simulink model "ex6_dvbs_chain_v2"  (R2022a)
settings: Solver=VariableStepAuto  StartTime=0.0  StopTime=1  RelTol=1e-3
values from neighbouring files (symbols this model uses):
  M = 4    [ex6_parameters.m]
  PS_beta = 0.35    [ex6_parameters.m]
  PS_osf = 10    [ex6_parameters.m]
  PS_span = 8    [ex6_parameters.m]
  Rb = 100e3    (= 100000)    [ex6_parameters.m]
libraries: commdigbbndpm3 x2, commfilt2 x2, commchan3 x1, commsink2 x1, commrandsrc3 x1, simulink x1
settings Model: Creator=E0624826  LastModifiedBy=Filippo
settings SolverCC: AlgebraicLoopSolver=TrustRegion
settings DebuggingCC: UnconnectedInputMsg=warning  UnconnectedOutputMsg=warning  UnconnectedLineMsg=warning  SFMachineParentedDataDiag=warning

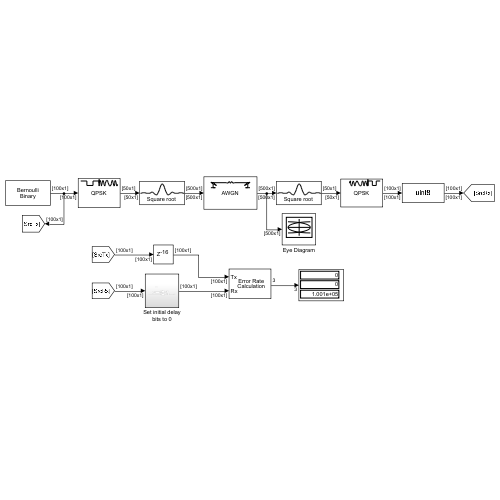
[thumbnail: Simulink's stored preview of the top-level diagram]
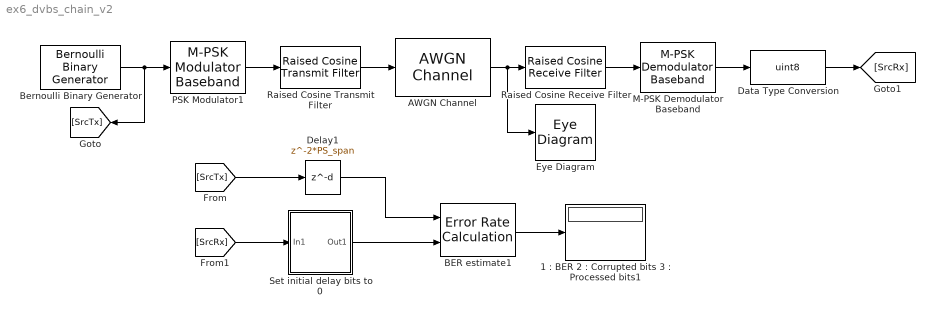
== system ex6_dvbs_chain_v2 ==
  "1 : BER 2 : Corrupted bits 3 : Processed bits1" : Display
  AWGN Channel : commchan3/AWGN Channel  InputProcessing=Columns as channels (frame based)  seed=randi(500)  noiseMode="Signal to noise ratio  (SNR)"  EbNodB=100  EsNodB=10  SNRdB=CHA_SNR  bitsPerSym=log2(M)  Ps=1  Tsym=Rs  variance=1
  BER estimate1 : commsink2/Error Rate Calculation  N=0  st_delay=0  cp_mode=Entire frame  subframe=[]  PMode=Port  WsName=ErrorVec  RsMode2=off  stop=off  numErr=100  maxBits=1e6
  Bernoulli Binary Generator : commrandsrc3/Bernoulli Binary Generator  ProbabilityOfZero=0.5  SeedSource=Auto  Seed=0  SampleTime=1/Rb  SamplesPerFrame=100  OutputDataType=uint8  SimulateUsing=Interpreted execution
  Data Type Conversion : DataTypeConversion  OutDataTypeStr=uint8  SaturateOnIntegerOverflow=off  RndMeth=Floor
  Delay1 : Delay  DelayLength=2*PS_span  InitialCondition=0  InputProcessing=Columns as channels (frame based)
  Eye Diagram : EyeDiagram
  M-PSK Demodulator Baseband : commdigbbndpm3/M-PSK Demodulator Baseband  M=M  OutType=Bit  DecType=Hard decision  VarSource=Dialog  Variance=1  Dec=Gray  Mapping=[0:7]  Ph=pi/M  outDtype1=Inherit via internal rule  outDtype2=Inherit via internal rule  derotateFactorWordLen=16  derotateFactorDataTypeStr=Inherit: Same word length as input  derotateFactorLastDataTypeStr=Inherit: Same word length as input
  PSK Modulator1 : commdigbbndpm3/M-PSK Modulator Baseband  M=M  InType=Bit  Enc=Gray  Mapping=[0:7]  Ph=pi/M  outDtype=double  outWordLen=16  outUDDataType=sfix(16)  outFracLenMode=Best precision  outFracLen=15  outDataTypeStr=double  outLastDataTypeStr=double
  Raised Cosine Receive Filter : commfilt2/Raised Cosine Receive Filter  filtType=Square root  R=PS_beta  filtSpan=PS_span  N=PS_osf  downFactor=PS_osf  downOffset=0  filterGain=1  InputProcessing=Columns as channels (frame based)  RateOptions=Enforce single-rate processing  framing=Mute  checkCoeff=off  variableName=rcRxFilt  currentFiltSpan=PS_span  D=(PS_span)/2  inputOffset=0  sampMode=Mute  saveAsFlag=0  rateMode=Downsampling  checkGain=Normalized  launchFVT=on  roundingMode=Floor  overflowMode=off  coeffDataTypeStr=Inherit: Same word length as input  coeffMin=[]  coeffMax=[]  coeffLastDataTypeStr=Inherit: Same word length as input  accumDataTypeStr=Inherit: Same as product output  accumLastDataTypeStr=Inherit: Same as product output  outputDataTypeStr=Inherit: Same as accumulator  outputMin=[]  outputMax=[]  outputLastDataTypeStr=Inherit: Same as accumulator
  Raised Cosine Transmit Filter : commfilt2/Raised Cosine Transmit Filter  filtType=Square root  R=PS_beta  filtSpan=PS_span  N=PS_osf  filterGain=1  InputProcessing=Columns as channels (frame based)  RateOptions=Enforce single-rate processing  framing=Mute  checkCoeff=off  variableName=rcTxFilt  checkGain=Normalized  sampMode=Mute  saveAsFlag=0  currentFiltSpan=PS_span  D=(PS_span)/2  launchFVT=on  roundingMode=Floor  overflowMode=off  coeffDataTypeStr=Inherit: Same word length as input  coeffMin=[]  coeffMax=[]  coeffLastDataTypeStr=Inherit: Same word length as input  outputDataTypeStr=Inherit: Same as accumulator  outputMin=[]  outputMax=[]  outputLastDataTypeStr=Inherit: Same as accumulator
  Set initial delay bits to 0 : Subsystem
  wires:
  BER estimate1/1 -> "1 : BER 2 : Corrupted bits 3 : Processed bits1"/1
  Bernoulli Binary Generator/1 -> PSK Modulator1/1, [SrcTx]
  M-PSK Demodulator Baseband/1 -> Data Type Conversion/1
  Data Type Conversion/1 -> [SrcRx]
  Raised Cosine Receive Filter/1 -> M-PSK Demodulator Baseband/1
  [SrcRx] -> Set initial delay bits to 0/1(In1)
  Set initial delay bits to 0/1(Out1) -> BER estimate1/2
  [SrcTx] -> Delay1/1
  Delay1/1 -> BER estimate1/1
  AWGN Channel/1 -> Eye Diagram/1, Raised Cosine Receive Filter/1
  Raised Cosine Transmit Filter/1 -> AWGN Channel/1
  PSK Modulator1/1 -> Raised Cosine Transmit Filter/1

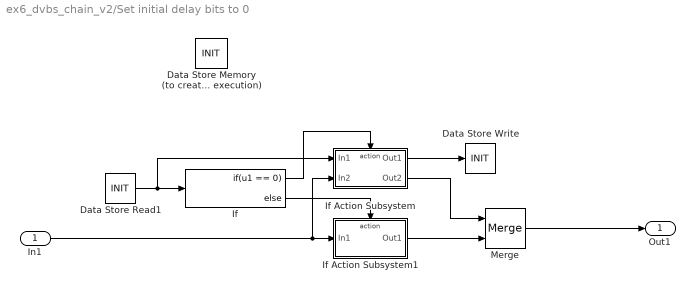
== system ex6_dvbs_chain_v2/Set initial delay bits to 0 ==
  In1 : Inport
  Data Store Memory (to create variable modifiable during execution) : DataStoreMemory  DataStoreName=INIT  ReadBeforeWriteMsg=warning  WriteAfterWriteMsg=warning  WriteAfterReadMsg=warning  ShowAdditionalParam=off
  Data Store Read1 : DataStoreRead  DataStoreName=INIT  IndexOptions=Index vector (dialog)  Indices=1  OutputSizes=1
  Data Store Write : DataStoreWrite  DataStoreName=INIT  IndexOptions=Index vector (dialog)  Indices=1  OutputSizes=1
  If : If  IfExpression=u1 == 0  ZeroCross=off
  If Action Subsystem : Subsystem  TreatAsAtomicUnit=on
  If Action Subsystem1 : Subsystem  TreatAsAtomicUnit=on
  Merge : Merge
  Out1 : Outport
  wires:
  Merge/1 -> Out1/1
  In1/1 -> If Action Subsystem/2(In2), If Action Subsystem1/1(In1)
  Data Store Read1/1 -> If Action Subsystem/1(In1), If/1
  If Action Subsystem/1(Out1) -> Data Store Write/1
  If Action Subsystem1/1(Out1) -> Merge/2
  If/2 -> If Action Subsystem1/Action
  If Action Subsystem/2(Out2) -> Merge/1
  If/1 -> If Action Subsystem/Action

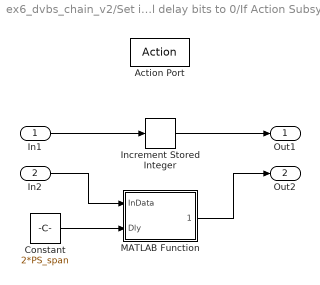
== system ex6_dvbs_chain_v2/Set initial delay bits to 0/If Action Subsystem ==
  In1 : Inport
  In2 : Inport  Port=2
  Action Port : ActionPort  ActionPortLabel=if(u1 == 0)
  Constant : Constant  Value=2*PS_span
  Increment Stored Integer : simulink/Additional Math & Discrete/Additional Math: Increment - Decrement/Increment Stored Integer
  MATLAB Function : MATLAB Function  TreatAsAtomicUnit=on
  Out1 : Outport
  Out2 : Outport  Port=2
  wires:
  In1/1 -> Increment Stored Integer/1
  Increment Stored Integer/1 -> Out1/1
  In2/1 -> MATLAB Function/1(InData)
  MATLAB Function/1(OutData) -> Out2/1
  Constant/1 -> MATLAB Function/2(Dly)

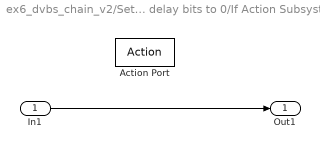
== system ex6_dvbs_chain_v2/Set initial delay bits to 0/If Action Subsystem1 ==
  In1 : Inport
  Action Port : ActionPort  ActionPortLabel=else
  Out1 : Outport
  wires:
  In1/1 -> Out1/1

== matlab function ex6_dvbs_chain_v2/Set initial delay bits to 0/If Action Subsystem/MATLAB Function ==
  data: InData input; OutData output; Dly input

function OutData = fcn( InData, Dly )
    OutData = uint8(zeros(length(InData),1));
    OutData(1+Dly:end) = InData(1+Dly:end);
end
